simulink model "statechart3"  (R2016b)
settings: Solver=VariableStepAuto  StartTime=0.0  StopTime=15  MaxStep=0.05  RelTol=1e-3
libraries: dspindex x2
settings Model: Creator=larry  LastModifiedBy=larry

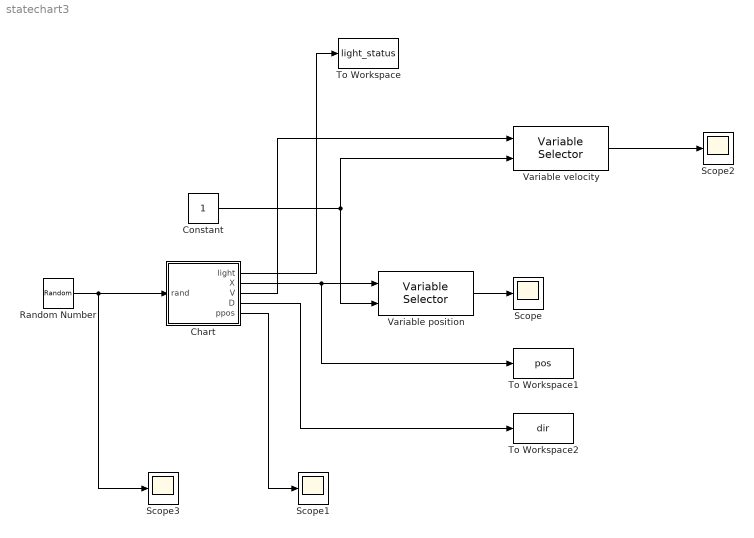
== system statechart3 ==
  Chart : Stateflow chart  TreatAsAtomicUnit=on
  Constant : Constant
  Random Number : RandomNumber  SampleTime=0.1
  Scope{,1..3} (4 alike) : Scope
  To Workspace : ToWorkspace  VariableName=light_status  SampleTime=-1
  To Workspace1 : ToWorkspace  VariableName=pos  SampleTime=-1
  To Workspace2 : ToWorkspace  VariableName=dir  SampleTime=-1
  Variable position : dspindex/Variable Selector  NumInputs=1  rowsOrCols=Columns  IdxMode=Variable  Elements=[1 3]  ZerOneIdxMode=One-based  errmode=Clip Index  FillMode=on  FillValues=0
  Variable velocity : dspindex/Variable Selector  NumInputs=1  rowsOrCols=Columns  IdxMode=Variable  Elements=[1 3]  ZerOneIdxMode=One-based  errmode=Clip Index  FillMode=on  FillValues=0
  wires:
  Chart/1(light) -> To Workspace/1
  Chart/2(X) -> To Workspace1/1, Variable position/1
  Constant/1 -> Variable position/2, Variable velocity/2
  Variable position/1 -> Scope/1
  Variable velocity/1 -> Scope2/1
  Chart/3(V) -> Variable velocity/1
  Chart/4(D) -> To Workspace2/1
  Chart/5(ppos) -> Scope1/1
  Random Number/1 -> Scope3/1, Chart/1(rand)

== stateflow chart statechart3/Chart ==
  note: Perception
  note: Decision
  note: Helper
  note: Action
  state Pedestrian1 [parallel]
    settings: executionOrder=3
    state Walking
      en:
      ppos = 0;
      du:
      ppos = temporalCount(sec);
      ex:
      ppos = 1;
    state Finish
    state Wait
    Walking -> Finish : after(1, sec)
    (default) -> Finish
    Wait -> Walking : [in(Light.G_R) && ...
        | Light.remain > 1]
    Finish -> Wait : [rand > THRES]
  state Light [parallel]
    settings: executionOrder=1
    state Y_R
      en:
      light = 4;
    state G_R
      en:
      light = 3;
      remain = G_LEN;
      du:
      remain = ...
      G_LEN-temporalCount(sec)
      ex:
      remain = 0;
    state R_G
      en:
      light = 1;
      remain = G_LEN;
      du:
      remain = ...
      G_LEN-temporalCount(sec);
      ex:
      remain = 0;
    state R_Y
      en:
      light = 2;
    G_R -> Y_R : after(G_LEN, sec)
    Y_R -> R_G : after(Y_LEN, sec)
    (default) -> R_G
    R_G -> R_Y : after(G_LEN, sec)
    R_Y -> G_R : after(Y_LEN, sec)
  state dummy [parallel]
    settings: executionOrder=2
    state RoadIntersection
      state Follow
        en:
        front = getFrontCarIdx(this);
        ex:
        front = uint8(0);
        state FollowFront
          du:
          followFrontCar(this, front, A_MAX);
        state FollowToStop
          state SlowDown
            en:
            updateBrakeAcc(this,A_MAX, ...
            closestObj(this,INTER,X(front,:)));
            du:
            accDrive(this);
          state Adjust
            du:
            adjustBehind(this, X(front,:), ...
            SAFE_DIST);
          (default) -> dummy.RoadIntersection.Follow.FollowToStop.SlowDown
          dummy.RoadIntersection.Follow.FollowToStop.SlowDown -> dummy.RoadIntersection.Follow.FollowToStop.Adjust : [isStopped(this)]
        (default) -> FollowFront [order 1] : [in(Light.G_R)]
        (junction 3047) -> FollowFront [order 2]
        (default) -> (junction 3047) [order 2]
        FollowFront -> (junction 3047) : [in(Light.Y_R)]
        (junction 3047) -> FollowToStop [order 1] : [stoppable(this, A_MAX,...
            | closestObj(this, INTER,X(front,:)))]
        FollowToStop -> FollowFront : [in(Light.G_R)]
      state FreeDriving
        state SlowToStop
          state SlowDown
            en:
            updateBrakeAcc(this,A_MAX,INTER);
            du:
            accDrive(this);
          state Stop
            en:
            A(this,:) = [0, 0];
            V(this,:) = [0, 0];
          state Adjust
            en:
            fixRate(this,V_MIN);
            du:
            adjustBehind(this,INTER,...
            SAFE_DIST);
          (default) -> dummy.RoadIntersection.FreeDriving.SlowToStop.SlowDown
          dummy.RoadIntersection.FreeDriving.SlowToStop.SlowDown -> dummy.RoadIntersection.FreeDriving.SlowToStop.Stop : [isStopped(this)]
          dummy.RoadIntersection.FreeDriving.SlowToStop.Stop -> dummy.RoadIntersection.FreeDriving.SlowToStop.Adjust : [closeBehind(this,INTER,...
              | SAFE_DIST)]
          dummy.RoadIntersection.FreeDriving.SlowToStop.Adjust -> dummy.RoadIntersection.FreeDriving.SlowToStop.Stop : [isStopped(this)]
        state RushToPass
          state Acc
            en:
            A(this,:) = D(this, :)*A_MAX;
            du:
            accDrive(this);
          state FixRate
            en:
            A(this,:) = [0, 0];
            du:
            fixRateDrive(this);
          (default) -> dummy.RoadIntersection.FreeDriving.RushToPass.Acc [order 2]
          dummy.RoadIntersection.FreeDriving.RushToPass.Acc -> dummy.RoadIntersection.FreeDriving.RushToPass.FixRate : [reachRate(this, V_MAX)]
          (default) -> dummy.RoadIntersection.FreeDriving.RushToPass.FixRate [order 1] : [reachRate(this,V_MAX)]
        state Normal
          state Acc
            en:
            A(this,:) = D(this, :)*A_MAX;
            du:
            accDrive(this);
          state FixRate
            en:
            A(this,:) = [0, 0];
            du:
            fixRateDrive(this);
          (default) -> dummy.RoadIntersection.FreeDriving.Normal.Acc [order 2]
          dummy.RoadIntersection.FreeDriving.Normal.Acc -> dummy.RoadIntersection.FreeDriving.Normal.FixRate : [reachRate(this, V_MAX)]
          (default) -> dummy.RoadIntersection.FreeDriving.Normal.FixRate [order 1] : [reachRate(this,V_MAX)]
        (default) -> (junction 3061) [order 1] : [~isGreen(this)]
        (junction 3061) -> dummy.RoadIntersection.FreeDriving.SlowToStop [order 1] : [stoppable(this,...
            | A_MAX,INTER)]
        (junction 3061) -> dummy.RoadIntersection.FreeDriving.RushToPass [order 2]
        dummy.RoadIntersection.FreeDriving.Normal -> (junction 3061) : [isYellow(this)]
        (default) -> dummy.RoadIntersection.FreeDriving.Normal [order 2]
        dummy.RoadIntersection.FreeDriving.SlowToStop -> dummy.RoadIntersection.FreeDriving.Normal : [isGreen(this)]
      (default) -> dummy.RoadIntersection.Follow [order 1] : [hasFrontCar(this, front)]
      dummy.RoadIntersection.FreeDriving -> dummy.RoadIntersection.Follow : [hasFrontCar(this, front)]
      dummy.RoadIntersection.Follow -> dummy.RoadIntersection.FreeDriving : [~hasFrontCar(this, front)]
      (default) -> dummy.RoadIntersection.FreeDriving [order 2]
    state Straight
      state FreeDriving
        state AccFromStop
          en:
          A(this,:) = D(this, :)*A_MAX;
          du:
          accDrive(this);
        state FixRate
          en:
          A(this,:) = [0, 0];
          fixRate(this, V_MAX);
          du:
          fixRateDrive(this);
        (default) -> dummy.Straight.FreeDriving.AccFromStop [order 2]
        (default) -> dummy.Straight.FreeDriving.FixRate [order 1] : [reachRate(this,V_MAX)]
        dummy.Straight.FreeDriving.AccFromStop -> dummy.Straight.FreeDriving.FixRate : [reachRate(this, V_MAX)]
      state Follow
        en:
        front = getFrontCarIdx(this);
        du:
        followFrontCar(this, front, A_MAX);
        ex:
        front = uint8(0);
      (default) -> dummy.Straight.FreeDriving
      dummy.Straight.FreeDriving -> dummy.Straight.Follow : [hasFrontCar(this, front)]
      dummy.Straight.Follow -> dummy.Straight.FreeDriving : [~hasFrontCar(this, front)]
    state IDLE
    state Turn
      en:
      turnFinished = false;
      state Right
        en:
        theta = 0;
        [x0, vturn, d0, p0] = prepRightTurn(this, dtheta);
        du:
        [theta, turnFinished] = ...
        rightTurn(this, x0, d0, p0, vturn, theta, dtheta);
        ex:
        INTER = resumeFromRightTurn(this, d0, vturn);
      state Left
        en:
        theta = 0;
        [x0, vturn, d0, p0] = prepLeftTurn(this, dtheta);
        du:
        [theta, turnFinished] = ...
        leftTurn(this, x0, d0, p0, vturn, theta, dtheta);
        ex:
        INTER = resumeFromLeftTurn(this, d0, vturn);
      (default) -> dummy.Turn.Right [order 1] : [decision == Decision.Right]
      (default) -> dummy.Turn.Left [order 2]
    (default) -> dummy.Straight [order 1] : [enabled]
    (default) -> dummy.IDLE [order 2]
    dummy.Straight -> dummy.RoadIntersection : [closeTo(this,INTER)]
    dummy.Turn -> dummy.Straight : [turnFinished]
    (junction 3015) -> dummy.Straight [order 1] : [decision == Decision.Straight]
    (junction 3015) -> dummy.Turn [order 2]
    dummy.RoadIntersection -> (junction 3015) : [~closeTo(this,INTER)]
  state Vehicle1 [parallel]
    settings: executionOrder=5
    state RoadIntersection
      state Follow
        en:
        front = getFrontCarIdx(this);
        ex:
        front = uint8(0);
        state NonStopFollow
          du:
          followFrontCar(this,front,A_MAX);
        state NormalFollow
          du:
          followFrontCar(this, front, A_MAX);
        state SlowToStop
          state SlowDown
            en:
            updateBrakeAcc(this,A_MAX, ...
            closestObj(this,INTER,X(front,:)));
            du:
            accDrive(this);
          state Adjust
            du:
            adjustBehind(this, X(front,:), ...
            SAFE_DIST);
          (default) -> Vehicle1.RoadIntersection.Follow.SlowToStop.SlowDown
          Vehicle1.RoadIntersection.Follow.SlowToStop.SlowDown -> Vehicle1.RoadIntersection.Follow.SlowToStop.Adjust : [isStopped(this)]
        (default) -> Vehicle1.RoadIntersection.Follow.NormalFollow [order 2]
        Vehicle1.RoadIntersection.Follow.NormalFollow -> (junction 3252) : [isYellow(this)]
        Vehicle1.RoadIntersection.Follow.SlowToStop -> Vehicle1.RoadIntersection.Follow.NormalFollow : [isGreen(this)]
        (junction 3252) -> Vehicle1.RoadIntersection.Follow.NonStopFollow [order 2]
        (default) -> (junction 3252) [order 1] : [~isGreen(this)]
        (junction 3252) -> Vehicle1.RoadIntersection.Follow.SlowToStop [order 1] : [stoppable(this, A_MAX,...
            | closestObj(this, INTER,X(front,:)))]
      state FreeDriving
        state RushToPass
          state Acc
            en:
            A(this,:) = D(this, :)*A_MAX;
            du:
            accDrive(this);
          state FixRate
            en:
            A(this,:) = [0, 0];
            du:
            fixRateDrive(this);
          (default) -> Vehicle1.RoadIntersection.FreeDriving.RushToPass.Acc [order 2]
          Vehicle1.RoadIntersection.FreeDriving.RushToPass.Acc -> Vehicle1.RoadIntersection.FreeDriving.RushToPass.FixRate : [reachRate(this, V_MAX)]
          (default) -> Vehicle1.RoadIntersection.FreeDriving.RushToPass.FixRate [order 1] : [reachRate(this,V_MAX)]
        state SlowToStop
          state SlowDown
            en:
            updateBrakeAcc(this,A_MAX,INTER);
            du:
            accDrive(this);
          state Stop
            en:
            A(this,:) = [0, 0];
            V(this,:) = [0, 0];
          (default) -> Vehicle1.RoadIntersection.FreeDriving.SlowToStop.SlowDown
          Vehicle1.RoadIntersection.FreeDriving.SlowToStop.SlowDown -> Vehicle1.RoadIntersection.FreeDriving.SlowToStop.Stop : [isStopped(this)]
        state Normal
          state Acc
            en:
            A(this,:) = D(this, :)*A_MAX;
            du:
            accDrive(this);
          state FixRate
            en:
            A(this,:) = [0, 0];
            du:
            fixRateDrive(this);
          (default) -> Vehicle1.RoadIntersection.FreeDriving.Normal.Acc [order 2]
          Vehicle1.RoadIntersection.FreeDriving.Normal.Acc -> Vehicle1.RoadIntersection.FreeDriving.Normal.FixRate : [reachRate(this, V_MAX)]
          (default) -> Vehicle1.RoadIntersection.FreeDriving.Normal.FixRate [order 1] : [reachRate(this,V_MAX)]
        (default) -> (junction 3267) [order 1] : [~isGreen(this)]
        (junction 3267) -> Vehicle1.RoadIntersection.FreeDriving.SlowToStop [order 1] : [stoppable(this,...
            | A_MAX,INTER)]
        (junction 3267) -> Vehicle1.RoadIntersection.FreeDriving.RushToPass [order 2]
        Vehicle1.RoadIntersection.FreeDriving.Normal -> (junction 3267) : [isYellow(this)]
        (default) -> Vehicle1.RoadIntersection.FreeDriving.Normal [order 2]
        Vehicle1.RoadIntersection.FreeDriving.SlowToStop -> Vehicle1.RoadIntersection.FreeDriving.Normal : [isGreen(this)]
      (default) -> Vehicle1.RoadIntersection.Follow [order 1] : [hasFrontCar(this, front)]
      Vehicle1.RoadIntersection.FreeDriving -> Vehicle1.RoadIntersection.Follow : [hasFrontCar(this, front)]
      Vehicle1.RoadIntersection.Follow -> Vehicle1.RoadIntersection.FreeDriving : [~hasFrontCar(this, front)]
      (default) -> Vehicle1.RoadIntersection.FreeDriving [order 2]
    state Straight
      state FreeDriving
        state FixRate
          en:
          A(this,:) = [0, 0];
          fixRate(this, V_MAX);
          du:
          fixRateDrive(this);
        state AccFromStop
          en:
          A(this,:) = D(this, :)*A_MAX;
          du:
          accDrive(this);
        (default) -> Vehicle1.Straight.FreeDriving.FixRate [order 1] : [reachRate(this,V_MAX)]
        Vehicle1.Straight.FreeDriving.AccFromStop -> Vehicle1.Straight.FreeDriving.FixRate : [reachRate(this, V_MAX)]
        (default) -> Vehicle1.Straight.FreeDriving.AccFromStop [order 2]
      state Follow
        en:
        front = getFrontCarIdx(this);
        du:
        followFrontCar(this, front, A_MAX);
        ex:
        front = uint8(0);
      (default) -> Vehicle1.Straight.FreeDriving
      Vehicle1.Straight.FreeDriving -> Vehicle1.Straight.Follow : [hasFrontCar(this, front)]
      Vehicle1.Straight.Follow -> Vehicle1.Straight.FreeDriving : [~hasFrontCar(this, front)]
    state IDLE
    state Turn
      en:
      turnFinished = false;
      state Right
        en:
        theta = 0;
        [x0, vturn, d0, p0] = prepRightTurn(this, dtheta);
        du:
        [theta, turnFinished] = ...
        rightTurn(this, x0, d0, p0, vturn, theta, dtheta);
        ex:
        INTER = resumeFromRightTurn(this, d0, vturn);
      state Left
        en:
        theta = 0;
        [x0, vturn, d0, p0] = prepLeftTurn(this, dtheta);
        du:
        [theta, turnFinished] = ...
        leftTurn(this, x0, d0, p0, vturn, theta, dtheta);
        ex:
        INTER = resumeFromLeftTurn(this, d0, vturn);
      (default) -> Vehicle1.Turn.Right [order 1] : [decision == Decision.Right]
      (default) -> Vehicle1.Turn.Left [order 2]
    (default) -> Vehicle1.Straight [order 1] : [enabled]
    (default) -> Vehicle1.IDLE [order 2]
    Vehicle1.Straight -> Vehicle1.RoadIntersection : [closeTo(this,INTER)]
    Vehicle1.Turn -> Vehicle1.Straight : [turnFinished]
    (junction 3238) -> Vehicle1.Straight [order 1] : [decision == Decision.Straight]
    (junction 3238) -> Vehicle1.Turn [order 2]
    Vehicle1.RoadIntersection -> (junction 3238) : [~closeTo(this,INTER)]
  state Vehicle2 [parallel]
    settings: executionOrder=4
    state RoadIntersection
      state Follow
        en:
        front = getFrontCarIdx(this);
        ex:
        front = uint8(0);
        state NonStopFollow
          du:
          followFrontCar(this,front,A_MAX);
        state NormalFollow
          du:
          followFrontCar(this, front, A_MAX);
        state SlowToStop
          state SlowDown
            en:
            updateBrakeAcc(this,A_MAX, ...
            closestObj(this,INTER,X(front,:)));
            du:
            accDrive(this);
          state Adjust
            du:
            adjustBehind(this, X(front,:), ...
            SAFE_DIST);
          (default) -> Vehicle2.RoadIntersection.Follow.SlowToStop.SlowDown
          Vehicle2.RoadIntersection.Follow.SlowToStop.SlowDown -> Vehicle2.RoadIntersection.Follow.SlowToStop.Adjust : [isStopped(this)]
        (default) -> Vehicle2.RoadIntersection.Follow.NormalFollow [order 2]
        Vehicle2.RoadIntersection.Follow.NormalFollow -> (junction 3153) : [isYellow(this)]
        Vehicle2.RoadIntersection.Follow.SlowToStop -> Vehicle2.RoadIntersection.Follow.NormalFollow : [isGreen(this)]
        (junction 3153) -> Vehicle2.RoadIntersection.Follow.NonStopFollow [order 2]
        (default) -> (junction 3153) [order 1] : [~isGreen(this)]
        (junction 3153) -> Vehicle2.RoadIntersection.Follow.SlowToStop [order 1] : [stoppable(this, A_MAX,...
            | closestObj(this, INTER,X(front,:)))]
      state FreeDriving
        state RushToPass
          state Acc
            en:
            A(this,:) = D(this, :)*A_MAX;
            du:
            accDrive(this);
          state FixRate
            en:
            A(this,:) = [0, 0];
            du:
            fixRateDrive(this);
          (default) -> Vehicle2.RoadIntersection.FreeDriving.RushToPass.Acc [order 2]
          Vehicle2.RoadIntersection.FreeDriving.RushToPass.Acc -> Vehicle2.RoadIntersection.FreeDriving.RushToPass.FixRate : [reachRate(this, V_MAX)]
          (default) -> Vehicle2.RoadIntersection.FreeDriving.RushToPass.FixRate [order 1] : [reachRate(this,V_MAX)]
        state SlowToStop
          state SlowDown
            en:
            updateBrakeAcc(this,A_MAX,INTER);
            du:
            accDrive(this);
          state Stop
            en:
            A(this,:) = [0, 0];
            V(this,:) = [0, 0];
          (default) -> Vehicle2.RoadIntersection.FreeDriving.SlowToStop.SlowDown
          Vehicle2.RoadIntersection.FreeDriving.SlowToStop.SlowDown -> Vehicle2.RoadIntersection.FreeDriving.SlowToStop.Stop : [isStopped(this)]
        state Normal
          state Acc
            en:
            A(this,:) = D(this, :)*A_MAX;
            du:
            accDrive(this);
          state FixRate
            en:
            A(this,:) = [0, 0];
            du:
            fixRateDrive(this);
          (default) -> Vehicle2.RoadIntersection.FreeDriving.Normal.Acc [order 2]
          Vehicle2.RoadIntersection.FreeDriving.Normal.Acc -> Vehicle2.RoadIntersection.FreeDriving.Normal.FixRate : [reachRate(this, V_MAX)]
          (default) -> Vehicle2.RoadIntersection.FreeDriving.Normal.FixRate [order 1] : [reachRate(this,V_MAX)]
        (default) -> (junction 3167) [order 1] : [~isGreen(this)]
        (junction 3167) -> Vehicle2.RoadIntersection.FreeDriving.SlowToStop [order 1] : [stoppable(this,...
            | A_MAX,INTER)]
        (junction 3167) -> Vehicle2.RoadIntersection.FreeDriving.RushToPass [order 2]
        Vehicle2.RoadIntersection.FreeDriving.Normal -> (junction 3167) : [isYellow(this)]
        (default) -> Vehicle2.RoadIntersection.FreeDriving.Normal [order 2]
        Vehicle2.RoadIntersection.FreeDriving.SlowToStop -> Vehicle2.RoadIntersection.FreeDriving.Normal : [isGreen(this)]
      (default) -> Vehicle2.RoadIntersection.Follow [order 1] : [hasFrontCar(this, front)]
      Vehicle2.RoadIntersection.FreeDriving -> Vehicle2.RoadIntersection.Follow : [hasFrontCar(this, front)]
      Vehicle2.RoadIntersection.Follow -> Vehicle2.RoadIntersection.FreeDriving : [~hasFrontCar(this, front)]
      (default) -> Vehicle2.RoadIntersection.FreeDriving [order 2]
    state Straight
      state FreeDriving
        state AccFromStop
          en:
          A(this,:) = D(this, :)*A_MAX;
          du:
          accDrive(this);
        state FixRate
          en:
          A(this,:) = [0, 0];
          fixRate(this, V_MAX);
          du:
          fixRateDrive(this);
        (default) -> Vehicle2.Straight.FreeDriving.AccFromStop [order 2]
        (default) -> Vehicle2.Straight.FreeDriving.FixRate [order 1] : [reachRate(this,V_MAX)]
        Vehicle2.Straight.FreeDriving.AccFromStop -> Vehicle2.Straight.FreeDriving.FixRate : [reachRate(this, V_MAX)]
      state Follow
        en:
        front = getFrontCarIdx(this);
        du:
        followFrontCar(this, front, A_MAX);
        ex:
        front = uint8(0);
      (default) -> Vehicle2.Straight.FreeDriving
      Vehicle2.Straight.FreeDriving -> Vehicle2.Straight.Follow : [hasFrontCar(this, front)]
      Vehicle2.Straight.Follow -> Vehicle2.Straight.FreeDriving : [~hasFrontCar(this, front)]
    state IDLE
    state Turn
      en:
      turnFinished = false;
      state Right
        en:
        theta = 0;
        [x0, vturn, d0, p0] = prepRightTurn(this, dtheta);
        du:
        [theta, turnFinished] = ...
        rightTurn(this, x0, d0, p0, vturn, theta, dtheta);
        ex:
        INTER = resumeFromRightTurn(this, d0, vturn);
      state Left
        en:
        theta = 0;
        [x0, vturn, d0, p0] = prepLeftTurn(this, dtheta);
        du:
        [theta, turnFinished] = ...
        leftTurn(this, x0, d0, p0, vturn, theta, dtheta);
        ex:
        INTER = resumeFromLeftTurn(this, d0, vturn);
      (default) -> Vehicle2.Turn.Right [order 1] : [decision == Decision.Right]
      (default) -> Vehicle2.Turn.Left [order 2]
    (default) -> Vehicle2.Straight [order 1] : [enabled]
    (default) -> Vehicle2.IDLE [order 2]
    Vehicle2.Straight -> Vehicle2.RoadIntersection : [closeTo(this,INTER)]
    Vehicle2.Turn -> Vehicle2.Straight : [turnFinished]
    (junction 3139) -> Vehicle2.Straight [order 1] : [decision == Decision.Straight]
    (junction 3139) -> Vehicle2.Turn [order 2]
    Vehicle2.RoadIntersection -> (junction 3139) : [~closeTo(this,INTER)]
  data: THRES local double size=1 =2; G_LEN constant double =4; Y_LEN constant double =0.5; remain local double size=1; self function_input; amax function_input; obj function_input; self function_input; res function_output; index function_input; self function_input; res function_output; self function_input; idx function_output; self function_input; self function_input; res function_output; self function_input; amax function_input; obj function_input; res function_output; needSafeDist function_input; self function_input; rate function_input; self function_input; res function_output; self function_input; rate function_input; res function_output; self function_input; self function_input; res function_output; obj function_input; self function_input; obj1 function_input; pos function_output; obj2 function_input; self function_input; index function_input; amax function_input; self function_input; obj function_input; dist function_input; res function_output; theta local double size=1; dtheta constant double size=1 =10; p0 local double size=[1, 2]; x0 local double size=[1, 2]; d0 local double size=[1, 2]; vturn local double size=1; dtheta constant double size=1 =3.3; d0 local double size=[1, 2]; x0 local double size=[1, 2]; p0 local double size=[1, 2]; vturn local double size=1; theta local double size=1; this constant uint8 size=1 =1; V_MAX constant double size=1 =2.5; A_MAX constant double size=1 =2.5; INTER local double size=[1, 2] =[-1, -0.5]; enabled local boolean size=1 =false; front local uint8 size=1 =uint8(0); decision local Enum: Decision size=1 =Decision.Straight; turnFinished local boolean size=1 =true; theta local double size=1; dtheta constant double size=1 =10; p0 local double size=[1, 2]; x0 local double size=[1, 2]; d0 local double size=[1, 2]; vturn local double size=1; dtheta constant double size=1 =3.3; d0 local double size=[1, 2]; x0 local double size=[1, 2]; p0 local double size=[1, 2]; vturn local double size=1; theta local double size=1; this constant uint8 size=1 =1; V_MAX constant double size=1 =2.5; A_MAX constant double size=1 =2.5; INTER local double size=[1, 2] =[-1, -0.5]; enabled local boolean size=1 =true; front local uint8 size=1 =uint8(0); decision local Enum: Decision size=1 =Decision.Straight; turnFinished local boolean size=1 =true; theta local double size=1; dtheta constant double size=1 =10; p0 local double size=[1, 2]; x0 local double size=[1, 2]; d0 local double size=[1, 2]; vturn local double size=1; dtheta constant double size=1 =3.3; d0 local double size=[1, 2]; x0 local double size=[1, 2]; p0 local double size=[1, 2]; vturn local double size=1; theta local double size=1; this constant uint8 size=1 =2; V_MAX constant double size=1 =2.5; A_MAX constant double size=1 =2.5; INTER local double size=[1, 2] =[-1, -0.5]; enabled local boolean size=1 =true; front local uint8 size=1 =uint8(0); decision local Enum: Decision size=1 =Decision.Right; turnFinished local boolean size=1 =true; self function_input; pos function_input; dist function_input; x0 function_output; vturn function_output; d0 function_output; p0 function_output; self function_input; dth function_input; self function_input; thf function_output; x0 function_input; d0 function_input; p0 function_input; vturn function_input; thi function_input; dth function_input; res function_output; self function_input; d0 function_input; inter function_output; vturn function_input; self function_input; dth function_input; x0 function_output; vturn function_output; d0 function_output; p0 function_output; self function_input; x0 function_input; d0 function_input; p0 function_input; vturn function_input; thi function_input; dth function_input; thf function_output; res function_output; self function_input; d0 function_input; vturn function_input; inter function_output; dt constant double size=1 =0.05; light output size=1; WORLD_SIZE constant double size=1 =8; X output size=[2,2] =[-7 -0.5;-5 -0.5]; SAFE_DIST constant double size=1 =1; V output size=[2,2] =[0 0;0 0]; V_MIN constant double size=1 =0.25; D output size=[2,2] =[1 0;1 0]; CAR_SIZE local size=[2, 2] =[0.3, 0.4; 0.3, 0.4]; A local size=[2,2] =[0 0;0 0]; rand input; ppos output
  function updateBrakeAcc(self, amax, obj):
    | function updateBrakeAcc(self, amax, obj)
    | 
    | x = X(self, :);
    | v = V(self, :);
    | 
    | % add safe distance
    | dist = norm(obj - x) - SAFE_DIST;
    | 
    | assert(dist >= 0);
    | 
    | vnorm = norm(v);
    | reverse = v/vnorm*(-1);
    | a = reverse*vnorm*vnorm/2/dist;
    | anorm = norm(a);
    | 
    | if(anorm >= amax)
    |     a = a/anorm*amax;
    | end
    | 
    | A(self, :) = a;
  function res = hasFrontCar(self, index):
    | function res = hasFrontCar(self, index)
    | 
    | if index == uint8(0)
    |     threshold = 1.8*SAFE_DIST;
    | else
    |     threshold = 2.2*SAFE_DIST;
    | end
    | 
    | FAR_AWAY = 100;
    | res = false;
    | num = size(X, 1);
    | if num == 1
    |     return;
    | end
    | 
    | dX = zeros(num, 1);
    | x = X(self,:);
    | d = D(self,:);
    | car_sz = CAR_SIZE(self, :);
    | 
    | for k=1:length(dX)
    |     xdelta = X(k,:) - x;
    |     delta_p = dot(xdelta, d);               % parallel distance
    |     delta_v = norm(xdelta - (d * delta_p)); % vertical distance
    |     
    |     % vertical distance is larger than car width
    |     if delta_v < car_sz(1)
    |         dX(k) = delta_p;
    |     else
    |         dX(k) = FAR_AWAY;
    |     end
    |     
    | %     dX(k) = dot(xdelta, d);
    |     if dX(k) < 0
    |         dX(k) = dX(k) + 2*WORLD_SIZE;
    |     end
    | end
    | 
    | % set zero dX to a large enough value
    | dX(dX == 0) = FAR_AWAY;
    | close = min(dX);
    | 
    | if close <= threshold
    |     res = true;
    | end
  function res = isStopped(self):
    | function res = isStopped(self)
    | 
    | v = V(self,:);
    | d = D(self,:);
    | 
    | res = false;
    | if(dot(v, d) <= 0)
    |     res = true;
    | end
    | if norm(v) < V_MIN
    |     res = true;
    | end
  function idx = getFrontCarIdx(self):
    | function idx = getFrontCarIdx(self)
    | 
    | dX = zeros(size(X, 1), 1);
    | x = X(self,:);
    | v = V(self,:);
    | d = D(self,:);
    | 
    | for k=1:length(dX)
    |     dX(k) = dot(X(k,:) - x, d);
    |     if dX(k) < 0
    |         dX(k) = dX(k) + 2*WORLD_SIZE;
    |     end
    | end
    | 
    | % set zero dX to a large enough value
    | dX(dX == 0) = 100;
    | [~, idx] = min(dX);
    | idx = uint8(idx);
  function fixRateDrive(self):
    | function fixRateDrive(self)
    |  
    | x = X(self, :);
    | v = V(self, :);
    | 
    | x = x + v * dt;
    | 
    | % a rounded world
    | if x(1) > WORLD_SIZE
    |     x(1) = -WORLD_SIZE;
    | elseif x(1) < -WORLD_SIZE
    |     x(1) = WORLD_SIZE;
    | elseif x(2) > WORLD_SIZE
    |     x(2) = -WORLD_SIZE;
    | elseif x(2) < -WORLD_SIZE
    |     x(2) = WORLD_SIZE;
    | end
    | 
    | X(self, :) = x;
  function res = isGreen(self):
    | function res = isGreen(self)
    | 
    | res = false;
    | d = D(self, :);
    | horizon = (abs(d(1)) ~= 0);
    | vertical = (abs(d(2)) ~= 0);
    | 
    | if in(Light.G_R) && horizon
    |     res = true;
    | elseif in(Light.R_G) && vertical
    |     res = true;
    | end
  function res = stoppable(self, amax, obj, needSafeDist):
    | function res = stoppable(self, amax, obj, needSafeDist)
    | 
    | x = X(self, :);
    | v = V(self, :);
    | 
    | % if needSafeDist ~= uint8(0)
    | %     dist = norm(obj - x) - SAFE_DIST;
    | % else
    | %     dist = norm(obj - x);
    | % end
    | 
    | dist = norm(obj - x) - SAFE_DIST;
    | 
    | vnorm = norm(v);
    | brake_dist = vnorm*vnorm/2.0/amax;
    | 
    | res = (brake_dist <= dist);
  function fixRate(self, rate):
    | function fixRate(self, rate)
    |  
    | v = V(self, :);
    | d = D(self, :);
    | if norm(v) < V_MIN
    |     v = d * V_MIN;
    | else
    |     v = v/norm(v)*rate;
    | end
    | 
    | V(self, :) = v;
  function res = isYellow(self):
    | function res = isYellow(self)
    | 
    | res = false;
    | d = D(self, :);
    | horizon = (abs(d(1)) ~= 0);
    | vertical = (abs(d(2)) ~= 0);
    | 
    | if in(Light.Y_R) && horizon
    |     res = true;
    | elseif in(Light.R_Y) && vertical
    |     res = true;
    | end
  function res = reachRate(self, rate):
    | function res = reachRate(self, rate)
    | 
    | res = false;
    | if norm(V(self, :)) >= rate
    |     res = true;
    | end
  function accDrive(self):
    | function accDrive(self)
    | 
    | x = X(self, :);
    | v = V(self, :);
    | a = A(self, :);
    | 
    | x = x + v * dt + 0.5 * a * dt * dt;
    | v = v + a * dt;
    | 
    | % a rounded world
    | if x(1) > WORLD_SIZE
    |     x(1) = -WORLD_SIZE;
    | elseif x(1) < -WORLD_SIZE
    |     x(1) = WORLD_SIZE;
    | elseif x(2) > WORLD_SIZE
    |     x(2) = -WORLD_SIZE;
    | elseif x(2) < -WORLD_SIZE
    |     x(2) = WORLD_SIZE;
    | end
    | X(self, :) = x;
    | V(self, :) = v;
  function res = closeTo(self, obj):
    | function res = closeTo(self, obj)
    | 
    | x = X(self, :);
    | d = D(self, :);
    | 
    | res = false;
    | dist = dot(obj - x, d);
    | if dist > 0 && dist <= 2.5*SAFE_DIST
    |     res = true;
    | end
  function pos = closestObj(self, obj1, obj2):
    | function pos = closestObj(self, obj1, obj2)
    | 
    | x = X(self, :);
    | d = D(self, :);
    | 
    | offset = 2*WORLD_SIZE;
    | dX = zeros(2, 1);
    | dX(1) = mod(dot(obj1 - x, d) + offset, offset);
    | dX(2) = mod(dot(obj2 - x, d) + offset, offset);
    | 
    | [~, index] = min(dX);
    | if index == 1
    |     pos = obj1;
    | else
    |     pos = obj2;
    | end
  function followFrontCar(self, index, amax):
    | function followFrontCar(self, index, amax)
    | 
    | % dX = zeros(size(X, 1), 1);
    | x = X(self,:);
    | v = V(self,:);
    | d = D(self,:);
    | a = [0, 0];
    | 
    | xfront = X(index, :);
    | vfront = V(index, :);
    | vfrontnorm = dot(vfront, d);
    | 
    | dist = dot(xfront - x, d);
    | vnorm = norm(v);
    | 
    | if dist <= 2*SAFE_DIST 
    |     
    |     if vnorm >= vfrontnorm 
    |         vo = d * vfrontnorm;
    |         if dist <= 1.5*SAFE_DIST
    |             vo = 0.75*vo;
    |         elseif dist <= SAFE_DIST
    |             vo = 0.5*vo;
    |         end
    |     else
    |         if dist <= SAFE_DIST
    |             vo = d * (vnorm + (vfrontnorm - vnorm)*0.2);
    |         else
    |             vo = d * (vnorm + (vfrontnorm - vnorm)*0.4);
    |         end
    |     end
    |     
    |     ar = (vo - v) / dt;
    |     arnorm = norm(ar);
    |     if arnorm > amax
    |         ar = ar/arnorm * amax;
    |         x = x + v * dt + 0.5 * ar * dt * dt;
    |         v = v + ar * dt;
    |     else
    |         x = x + (v + vo) * dt / 2;
    |         v = vo;
    |     end
    |     a = ar;
    | else
    |     x = x + v * dt;
    | end
    | 
    | % a rounded world
    | if x(1) > WORLD_SIZE
    |     x(1) = -WORLD_SIZE;
    | elseif x(1) < -WORLD_SIZE
    |     x(1) = WORLD_SIZE;
    | elseif x(2) > WORLD_SIZE
    |     x(2) = -WORLD_SIZE;
    | elseif x(2) < -WORLD_SIZE
    |     x(2) = WORLD_SIZE;
    | end
    | 
    | X(self,:) = x;
    | V(self,:) = v;
    | A(self,:) = a;
  function res = closeBehind(self, obj, dist):
    | function res = closeBehind(self, obj, dist)
    | 
    | x = X(self, :);
    | d = D(self, :);
    | 
    | res = false;
    | diff = dot(obj - x, d);
    | if diff > dist && diff - dist <= 1.5*SAFE_DIST
    |     res = true;
    | end
  function adjustBehind(self, pos, dist):
    | function adjustBehind(self, pos, dist)
    | 
    | x = X(self,:);
    | v = V(self,:);
    | d = D(self,:);
    | 
    | % assert(norm(v) <= 1);
    | 
    | diff = dot(pos - x, d);
    | if diff > dist
    |     v = v/norm(v)*V_MIN;
    |     dxnorm = V_MIN * dt;
    |     if (diff - dxnorm) >= dist
    |         x = x + dxnorm * d;
    |     else
    |         x = pos - dist * d;
    |     end
    | else
    |     v = [0, 0];
    | end
    | 
    | X(self, :) = x;
    | V(self, :) = v;
  function [x0, vturn, d0, p0] = prepRightTurn(self, dth):
    | function [x0, vturn, d0, p0] = prepRightTurn(self, dth)
    | 
    | d0 = D(self, :);
    | vturn = 0.5 * deg2rad(dth) / dt;
    | 
    | if isequal(d0, [1 0])
    |     x0 = [-1 -0.5];
    |     p0 = [0 0.5];
    | elseif isequal(d0, [-1 0])
    |     x0 = [1 0.5];
    |     p0 = [0 -0.5];
    | elseif isequal(d0, [0 1])
    |     x0 = [0.5 -1];
    |     p0 = [-0.5 0];
    | elseif isequal(d0, [0 -1])
    |     x0 = [-0.5 1];
    |     p0 = [0.5 0];
    | else
    |     error('Unknown orientation');
    | end
  function [thf, res] = rightTurn(self, x0, d0, p0, vturn, thi, dth):
    | function [thf, res] = rightTurn(self, x0, d0, p0, vturn, thi, dth)
    | 
    | res = false;
    | thf = thi + dth;
    | rad = deg2rad(thf);
    | 
    | if thf > 90
    |     res = true;
    |     return;
    | end
    | 
    | rot = [cos(rad) sin(rad); -sin(rad) cos(rad)];
    | pf = (rot * p0')';
    | df = (rot * d0')';
    | 
    | diff = pf - p0;
    | 
    | X(self, :) = x0 + diff;
    | V(self, :) = df * vturn;
    | D(self, :) = df;
  function inter = resumeFromRightTurn(self, d0, vturn):
    | function inter = resumeFromRightTurn(self, d0, vturn)
    | 
    | if isequal(d0, [1 0])
    |     df = [0 -1];
    |     xf = [-0.5 -1];
    |     inter = [-0.5 1];
    | elseif isequal(d0, [-1 0])
    |     df = [0 1];
    |     xf = [0.5 1];
    |     inter = [-0.5 -1];
    | elseif isequal(d0, [0 1])
    |     df = [1 0];
    |     xf = [1 -0.5];
    |     inter = [-1 -0.5];
    | elseif isequal(d0, [0 -1])
    |     df = [-1 0];
    |     xf = [-1 0.5];
    |     inter = [1 0.5];
    | else
    |     error('Unknown orientation');
    | end
    | 
    | X(self, :) = xf;
    | V(self, :) = df * vturn;
    | D(self, :) = df;
  function [x0, vturn, d0, p0] = prepLeftTurn(self, dth):
    | function [x0, vturn, d0, p0] = prepLeftTurn(self, dth)
    |  
    | d0 = D(self, :);
    | vturn = 1.5 * deg2rad(dth) / dt;
    | 
    | if isequal(d0, [1 0])
    |     x0 = [-1 -0.5];
    |     p0 = [0 -1.5];
    | elseif isequal(d0, [-1 0])
    |     x0 = [1 0.5];
    |     p0 = [0 1.5];
    | elseif isequal(d0, [0 1])
    |     x0 = [0.5 -1];
    |     p0 = [1.5 0];
    | elseif isequal(d0, [0 -1])
    |     x0 = [-0.5 1];
    |     p0 = [-1.5 0];
    | else
    |     error('Unknown orientation');
    | end
  function [thf, res] = leftTurn(self, x0, d0, p0, vturn, thi, dth):
    | function [thf, res] = leftTurn(self, x0, d0, p0, vturn, thi, dth)
    | 
    | res = false;
    | thf = thi + dth;
    | rad = deg2rad(thf);
    | 
    | if thf > 90
    |     res = true;
    |     return;
    | end
    | 
    | rot = [cos(rad) -sin(rad); sin(rad) cos(rad)];
    | pf = (rot * p0')';
    | df = (rot * d0')';
    | 
    | diff = pf - p0;
    | 
    | X(self, :) = x0 + diff;
    | V(self, :) = df * vturn;
    | D(self, :) = df;
  function inter = resumeFromLeftTurn(self, d0, vturn):
    | function inter = resumeFromLeftTurn(self, d0, vturn)
    | 
    | if isequal(d0, [1 0])
    |     df = [0 1];
    |     xf = [0.5 1];
    |     inter = [0.5 -1];
    | elseif isequal(d0, [-1 0])
    |     df = [0 -1];
    |     xf = [-0.5 -1];
    |     inter = [-0.5 1];
    | elseif isequal(d0, [0 1])
    |     df = [-1 0];
    |     xf = [-1 0.5];
    |     inter = [-1 -0.5];
    | elseif isequal(d0, [0 -1])
    |     df = [1 0];
    |     xf = [1 -0.5];
    |     inter = [-1 0.5];
    | else
    |     error('Unknown orientation');
    | end
    | 
    | X(self, :) = xf;
    | V(self, :) = df * vturn;
    | D(self, :) = df;
